simulink model "Expriment_Emotion"  (R2014a)
settings: Solver=FixedStepDiscrete  SolverMode=SingleTasking  StartTime=0.0  StopTime=inf  FixedStep=0.01  RelTol=1e-3
PostLoadFcn:
  | h_RPStest = RPStest;
model workspace (MAT data in the model file):
  gtest = 0
undefined symbols (not defined in the file or in its folder): avert, avert_freq_factor, avert_gaze_dirs_chance, avert_gaze_duration_factor, avert_head_frequency_factor, avert_head_speed, BML, BML1, BML2, bmlsL, bmlsM, bodyBusyFlag, clock, emotion_amount_factor, faceBusyFlag, fileID, GAZE_WIN, gazing, mut_freq_factor, mutual_gaze_duration_factor, P, pose_cat_chance, pose_chanc_factor, pose_chance_factor, pose_frequency_factor, pose_lean, pose_lean_flag, pose_space, pose_speed, pose_twitch, pr, serial, STATE_BEFORE, STATE_GO, STATE_OVER, STATE_READY, Stateflow
libraries: simulink x24, instrumentlib x6, realtime_pacer_lib x2, lib_affectiveChar_behavior x1, lib_affectiveChar_input x1
(part 2 of 6)

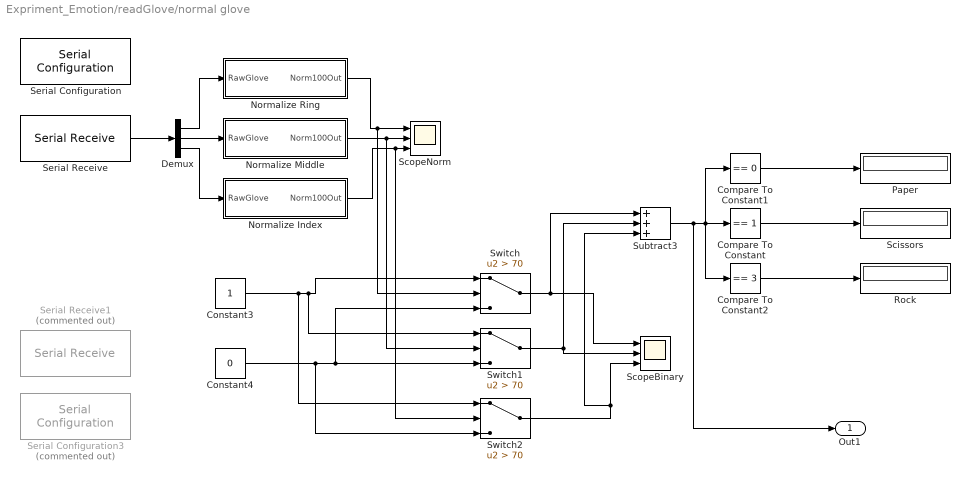
== system Expriment_Emotion/readGlove/normal glove ==
  Compare To Constant : simulink/Logic and Bit Operations/Compare To Constant  relop===  const=1  OutDataTypeStr=boolean
  Compare To Constant1 : simulink/Logic and Bit Operations/Compare To Constant  relop===  const=0  OutDataTypeStr=boolean
  Compare To Constant2 : simulink/Logic and Bit Operations/Compare To Constant  relop===  const=3  OutDataTypeStr=boolean
  Constant3 : Constant
  Constant4 : Constant  Value=0
  Demux : Demux  Outputs=3
  Normalize Index : Subsystem
  Normalize Middle : Subsystem
  Normalize Ring : Subsystem
  Paper : Display
  Rock : Display
  Scissors : Display
  ScopeBinary : Scope  NumInputPorts=3
      settings: YMin=-0.5~-0.5~-0.5  YMax=1.5~1.5~1.5
  ScopeNorm : Scope  NumInputPorts=3
      settings: TimeRange=10  YMin=-20~-20~-20  YMax=150~150~150
  Serial Configuration : instrumentlib/Serial Configuration  Priority=-200000  ComPortMenu=<Please select a port...>  ComPort=COM4  ObjConstructor=serial('COM4');  BaudRate=9600  DataBits=8  Parity=none  StopBits=1  FlowControl=none  Timeout=10  ByteOrder=LittleEndian
  Serial Configuration3 : instrumentlib/Serial Configuration  Priority=-200000  Commented=on  ComPortMenu=<Please select a port...>  ComPort=COM5  ObjConstructor=serial('COM5');  BaudRate=9600  DataBits=8  Parity=none  StopBits=1  FlowControl=none  Timeout=10  ByteOrder=LittleEndian
  Serial Receive : instrumentlib/Serial Receive  ComPortMenu=<Please select a port...>  ComPort=COM4  ObjConstructor=serial('COM4');  Terminator=<none>  DataSize="[3  1]"  DataType=uint8  EnableBlockingMode=on  ActionDataUnavailable=Output last received value  CustomValue=0  SampleTime=0.01
  Serial Receive1 : instrumentlib/Serial Receive  Commented=on  ComPortMenu=<Please select a port...>  ComPort=COM5  ObjConstructor=serial('COM5');  Terminator=<none>  DataSize="[3  1]"  DataType=uint8  EnableBlockingMode=on  ActionDataUnavailable=Output last received value  CustomValue=0  SampleTime=0.01
  Subtract3 : Sum  Inputs=+++
  Switch : Switch  Criteria=u2 > Threshold  Threshold=70
  Switch1 : Switch  Criteria=u2 > Threshold  Threshold=70
  Switch2 : Switch  Criteria=u2 > Threshold  Threshold=70
  Out1 : Outport
  wires:
  Demux/1 -> Normalize Ring/1(RawGlove)
  Demux/2 -> Normalize Middle/1(RawGlove)
  Demux/3 -> Normalize Index/1(RawGlove)
  Switch/1 -> ScopeBinary/1, Subtract3/1
  Constant3/1 -> Switch2/1, Switch1/1, Switch/1
  Constant4/1 -> Switch2/3, Switch1/3, Switch/3
  Switch1/1 -> ScopeBinary/2, Subtract3/2
  Switch2/1 -> Subtract3/3, ScopeBinary/3
  Subtract3/1 -> Compare To Constant/1, Compare To Constant2/1, Compare To Constant1/1, Out1/1
  Compare To Constant1/1 -> Paper/1
  Compare To Constant/1 -> Scissors/1
  Compare To Constant2/1 -> Rock/1
  Normalize Index/1(Norm100Out) -> Switch2/2, ScopeNorm/3
  Normalize Ring/1(Norm100Out) -> Switch/2, ScopeNorm/1
  Normalize Middle/1(Norm100Out) -> ScopeNorm/2, Switch1/2
  Serial Receive/1 -> Demux/1

== system Expriment_Emotion/readSHORE/smile ==
  In1 : Inport
  ifSmile : MATLAB Function  TreatAsAtomicUnit=on
  Out1 : Outport
  wires:
  ifSmile/1(y) -> Out1/1
  In1/1 -> ifSmile/1(u)

== system Expriment_Emotion/GazeFollowSubsystem/reactiveGaze/createGazePawn/sendBML ==
  In1 : Inport  OutDataTypeStr=double  PortDimensions=[1000 1]
  f : TriggerPort  TriggerType=function-call
      settings: CopyFcn=Stateflow.SLINSF.SimulinkMan.removeBlockPreDeleteFcn  PreDeleteFcn=Stateflow.SLINSF.SimulinkMan.unsafePredeleteFcn
  C++ S-Function2 : S-Function  FunctionName=yarpSendText_sfun  Parameters='/sim/out/bml8', '/SB/in/bml'  EnableBusSupport=off
  wires:
  In1/1 -> C++ S-Function2/1

== system Expriment_Emotion/GazeFollowSubsystem/reactiveGaze/createGazePawn/sendSBM ==
  In2 : Inport  OutDataTypeStr=double  PortDimensions=[1000 1]
  f : TriggerPort  TriggerType=function-call
      settings: CopyFcn=Stateflow.SLINSF.SimulinkMan.removeBlockPreDeleteFcn  PreDeleteFcn=Stateflow.SLINSF.SimulinkMan.unsafePredeleteFcn
  C++ S-Function2 : S-Function  FunctionName=yarpSendText_sfun  Parameters='/sim/out/smb5', '/SB/in/sbm'  EnableBusSupport=off
  wires:
  In2/1 -> C++ S-Function2/1
